simulink model "PrimeiraOrdemSeno"  (R2015a)
settings: Solver=ode5  StartTime=0.0  StopTime=4  FixedStep=0.00001  RelTol=1e-4
settings Model: Creator=user  LastModifiedBy=user
settings SolverCC: ZeroCrossAlgorithm=Adaptive

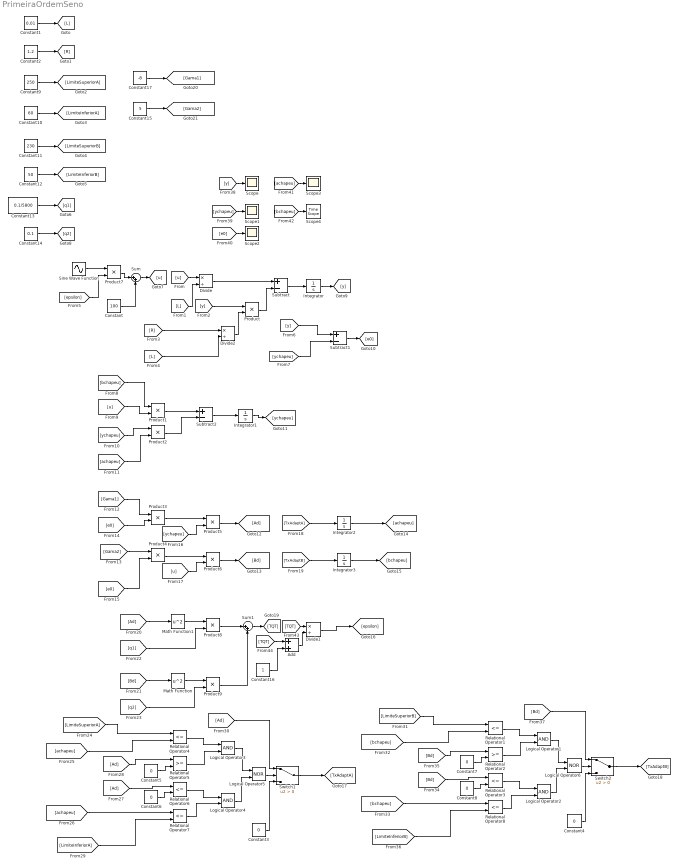
== system PrimeiraOrdemSeno ==
  Add : Sum
  Constant : Constant  Value=100
  Constant1 : Constant  Value=0.01
  Constant10 : Constant  Value=60
  Constant11 : Constant  Value=230
  Constant12 : Constant  Value=50
  Constant13 : Constant  Value=0.1/5800
  Constant14 : Constant  Value=0.1
  Constant15 : Constant  Value=5
  Constant16 : Constant
  Constant17 : Constant  Value=-8
  Constant2 : Constant  Value=1.2
  Constant{3..8} (6 alike) : Constant  Value=0
  Constant9 : Constant  Value=250
  Divide : Product  Inputs=*/
  Divide1 : Product  Inputs=*/
  Divide2 : Product  Inputs=*/
  Integrator : Integrator
  Integrator1 : Integrator
  Integrator2 : Integrator  InitialCondition=115
  Integrator3 : Integrator  InitialCondition=80
  Logical Operator{1..4} (4 alike) : Logic  AllPortsSameDT=off  OutDataTypeStr=boolean
  Logical Operator5 : Logic  Operator=NOR  AllPortsSameDT=off  OutDataTypeStr=boolean
  Logical Operator6 : Logic  Operator=NOR  AllPortsSameDT=off  OutDataTypeStr=boolean
  Math Function : Math  Operator=square  SaturateOnIntegerOverflow=on
  Math Function1 : Math  Operator=square  SaturateOnIntegerOverflow=on
  Product{,1..9} (10 alike) : Product
  Relational Operator{1,3..4,6..8} (6 alike) : RelationalOperator  Operator=<=  OutDataTypeStr=boolean
  Relational Operator2 : RelationalOperator  OutDataTypeStr=boolean
  Relational Operator5 : RelationalOperator  OutDataTypeStr=boolean
  Scope{,1..3} (4 alike) : Scope
      Scope settings: YMin=98  YMax=121
      Scope1 settings: YMin=72.5  YMax=102.5  SampleInput=on
      Scope2 settings: YMin=-0.6  YMax=0.55  SaveName=ScopeData2  SampleInput=on
      Scope3 settings: YMin=119.318  YMax=119.318  SaveName=ScopeData3  SampleInput=on
  Scope4 : TimeScope
  Sine Wave Function : Sin  Amplitude=100  Frequency=1000  SampleTime=0
  Subtract : Sum  Inputs=+-
  Subtract1 : Sum  Inputs=+-
  Subtract2 : Sum  Inputs=+-
  Sum : Sum  Inputs=|++
  Sum1 : Sum  Inputs=|++
  Switch1 : Switch  Criteria=u2 > Threshold
  Switch2 : Switch  Criteria=u2 > Threshold
  wires:
  Constant/1 -> Sum/2
  [L] -> Divide/2
  Divide2/1 -> Product/2
  [L] -> Divide2/2
  [R] -> Divide2/1
  Product/1 -> Subtract/2
  Divide/1 -> Subtract/1
  Subtract/1 -> Integrator/1
  Integrator/1 -> [y]
  [y] -> Product/1
  Sum/1 -> [u]
  [u] -> Divide/1
  [y] -> Subtract1/1
  [ychapeu] -> Subtract1/2
  Subtract1/1 -> [e0]
  Constant1/1 -> [L]
  Constant2/1 -> [R]
  Product1/1 -> Subtract2/1
  Subtract2/1 -> Integrator1/1
  Product2/1 -> Subtract2/2
  [achapeu] -> Product2/2
  [ychapeu] -> Product2/1
  [u] -> Product1/2
  [bchapeu] -> Product1/1
  Integrator1/1 -> [ychapeu]
  [e0] -> Product3/2
  [Gama1] -> Product3/1
  [Gama2] -> Product4/1
  [e0] -> Product4/2
  Product4/1 -> Product6/1
  Product3/1 -> Product5/1
  [ychapeu] -> Product5/2
  [u] -> Product6/2
  Product6/1 -> [Bd]
  Product5/1 -> [Ad]
  [TxAdaptA] -> Integrator2/1
  [TxAdaptB] -> Integrator3/1
  Integrator3/1 -> [bchapeu]
  Integrator2/1 -> [achapeu]
  Product7/1 -> Sum/1
  Sine Wave Function/1 -> Product7/1
  [epsilon] -> Product7/2
  [Bd] -> Math Function/1
  [Ad] -> Math Function1/1
  Math Function1/1 -> Product8/1
  Math Function/1 -> Product9/1
  [q1] -> Product8/2
  [q2] -> Product9/2
  Product9/1 -> Sum1/2
  Product8/1 -> Sum1/1
  Relational Operator6/1 -> Logical Operator4/1
  Relational Operator7/1 -> Logical Operator4/2
  Relational Operator5/1 -> Logical Operator3/2
  Relational Operator4/1 -> Logical Operator3/1
  Logical Operator3/1 -> Logical Operator5/1
  Logical Operator4/1 -> Logical Operator5/2
  Logical Operator5/1 -> Switch1/2
  [Ad] -> Switch1/1
  Constant3/1 -> Switch1/3
  Switch1/1 -> [TxAdaptA]
  [LimiteSuperiorA] -> Relational Operator4/1
  [LimiteInferiorA] -> Relational Operator7/2
  Constant6/1 -> Relational Operator6/2
  Constant5/1 -> Relational Operator5/2
  [Ad] -> Relational Operator6/1
  [Ad] -> Relational Operator5/1
  Constant9/1 -> [LimiteSuperiorA]
  Constant10/1 -> [LimiteInferiorA]
  Constant11/1 -> [LimiteSuperiorB]
  Constant12/1 -> [LimiteInferiorB]
  [achapeu] -> Relational Operator7/1
  [achapeu] -> Relational Operator4/2
  Constant13/1 -> [q1]
  Constant14/1 -> [q2]
  Relational Operator3/1 -> Logical Operator2/1
  Relational Operator8/1 -> Logical Operator2/2
  Relational Operator2/1 -> Logical Operator1/2
  Relational Operator1/1 -> Logical Operator1/1
  Logical Operator1/1 -> Logical Operator6/1
  Logical Operator2/1 -> Logical Operator6/2
  Logical Operator6/1 -> Switch2/2
  [Bd] -> Switch2/1
  Constant4/1 -> Switch2/3
  Switch2/1 -> [TxAdaptB]
  [LimiteSuperiorB] -> Relational Operator1/1
  [LimiteInferiorB] -> Relational Operator8/2
  Constant8/1 -> Relational Operator3/2
  Constant7/1 -> Relational Operator2/2
  [Bd] -> Relational Operator3/1
  [Bd] -> Relational Operator2/1
  [bchapeu] -> Relational Operator8/1
  [bchapeu] -> Relational Operator1/2
  [y] -> Scope/1
  [ychapeu] -> Scope1/1
  [e0] -> Scope2/1
  [achapeu] -> Scope3/1
  [bchapeu] -> Scope4/1
  Constant17/1 -> [Gama1]
  Constant15/1 -> [Gama2]
  Divide1/1 -> [epsilon]
  Add/1 -> Divide1/2
  Constant16/1 -> Add/2
  Sum1/1 -> [TQT]
  [TQT] -> Divide1/1
  [TQT] -> Add/1
